simulink model "test"  (Simulink 7.7)
settings: Solver=ode45  StartTime=0.0  StopTime=10.0  RelTol=1e-3
values from neighbouring files (symbols this model uses):
  BB = B_cruise    [parameter.m]
undefined symbols (not defined in the file or in its folder): dd
libraries: dspmtrx3 x2, dspinverses x1
settings Model: Creator=Li  LastModifiedBy=Li

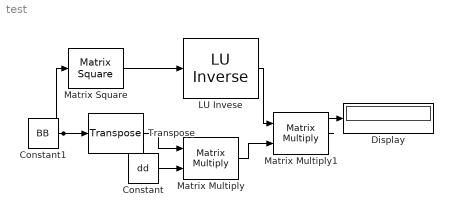
== system test ==
  " LU Invese" : dspinverses/ LU Inverse  SystemSampleTime=-1
  Constant : Constant  Value=dd
  Constant1 : Constant  Value=BB
  Display : Display
  Matrix Square : dspmtrx3/Matrix Square  SystemSampleTime=-1  OutMin=[]  OutMax=[]
  Matrix Multiply : Product  Multiplication=Matrix(*)
  Matrix Multiply1 : Product  Multiplication=Matrix(*)
  Transpose : dspmtrx3/Transpose  SystemSampleTime=-1  Hermitian=off  overflowFlag=off
  wires:
  Constant1/1 -> Transpose/1, Matrix Square/1
  Transpose/1 -> Matrix Multiply/1
  Constant/1 -> Matrix Multiply/2
  Matrix Multiply/1 -> Matrix Multiply1/2
  Matrix Square/1 -> " LU Invese"/1
  " LU Invese"/1 -> Matrix Multiply1/1
  Matrix Multiply1/1 -> Display/1
